simulink model "coupled_tanks"  (R2020a)
settings: Solver=ode45  StartTime=0.0  StopTime=1000  MaxStep=1e-1  RelTol=1e-3  EnableMultiTasking=on
settings Model: Creator=francesco  LastModifiedBy=啊包PC
settings DataIOCC: LimitDataPoints=on  SaveFormat=Array  ReturnWorkspaceOutputs=off
settings OptimizationCC: LifeSpan=inf
settings DebuggingCC: SFUnexpectedBacktrackingDiag=warning  SFNoUnconditionalDefaultTransitionDiag=warning  SFExecutionAtInitializationDiag=none  ArithmeticOperatorsInVariantConditions=warning
settings HardwareCC: ProdBitPerPointer=32  ProdBitPerSizeT=32  ProdBitPerPtrDiffT=32  ProdLargestAtomicFloat=None  ProdIntDivRoundTo=Undefined  ProdEndianess=Unspecified  ProdWordSize=32  ProdHWDeviceType=32-bit Generic
settings ModelReferenceCC: PropagateSignalLabelsOutOfModel=off
settings SFSimCC: SimUseLocalCustomCode=off  CustomCodeUndefinedFunction=UseInterfaceOnly
settings RTWCC: RTWUseLocalCustomCode=off
settings CodeAppCC: StateflowObjectComments=on
settings GRTTargetCC: TargetLangStandard=C89/C90 (ANSI)
settings ConfigComp: CovMetricSettings=dw  CovHtmlReporting=on  CovSaveCumulativeToWorkspaceVar=on  CovSaveSingleToWorkspaceVar=on  CovExternalEMLEnable=off

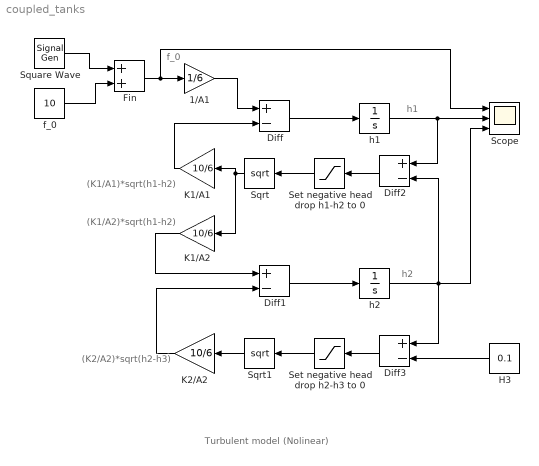
== system coupled_tanks ==
  note: (K1/A1)*sqrt(h1-h2)
  note: h1
  note: f_0
  note: h2
  note: (K1/A2)*sqrt(h1-h2)
  note: (K2/A2)*sqrt(h2-h3)
  note: Turbulent model (Nolinear)
  1/A1 : Gain  Gain=1/6
  Diff{,1..3} (4 alike) : Sum  Inputs=+-
  Fin : Sum
  H3 : Constant  Value=0.1
  K1/A1 : Gain  Gain=10/6
  K1/A2 : Gain  Gain=10/6
  K2/A2 : Gain  Gain=10/6
  Scope : Scope  NumInputPorts=3
  Set negative head drop h1-h2 to 0 : Saturate  UpperLimit=Inf  LowerLimit=0  ZeroCross=off
  Set negative head drop h2-h3 to 0 : Saturate  UpperLimit=Inf  LowerLimit=0  ZeroCross=off
  Sqrt : Sqrt  SaturateOnIntegerOverflow=on
  Sqrt1 : Sqrt  SaturateOnIntegerOverflow=on
  Square Wave : SignalGenerator  WaveForm=square  Amplitude=0.3*10  Frequency=1/60
  f_0 : Constant  Value=10
  h1 : Integrator
  h2 : Integrator
  wires:
  Square Wave/1 -> Fin/1
  f_0/1 -> Fin/2
  1/A1/1 -> Diff/1
  Diff/1 -> h1/1
  h1/1 -> Scope/2, Diff2/1
  Fin/1 -> Scope/1, 1/A1/1
  h2/1 -> Diff3/1, Diff2/2, Scope/3
  Diff2/1 -> Set negative head drop h1-h2 to 0/1
  Set negative head drop h1-h2 to 0/1 -> Sqrt/1
  Sqrt/1 -> K1/A2/1, K1/A1/1
  K1/A1/1 -> Diff/2
  Diff1/1 -> h2/1
  K1/A2/1 -> Diff1/1
  Diff3/1 -> Set negative head drop h2-h3 to 0/1
  Set negative head drop h2-h3 to 0/1 -> Sqrt1/1
  Sqrt1/1 -> K2/A2/1
  H3/1 -> Diff3/2
  K2/A2/1 -> Diff1/2
